simulink model "Validacion"  (R2022b)
settings: Solver=VariableStepAuto  StartTime=0.0  StopTime=10  RelTol=1e-3
values from neighbouring files (symbols this model uses):
  tt = tr-tr(1)    [LAB.m]
  ut = ur-u(pos(1)-1)    [LAB.m]
settings Model: Creator=emanu  LastModifiedBy=emanu

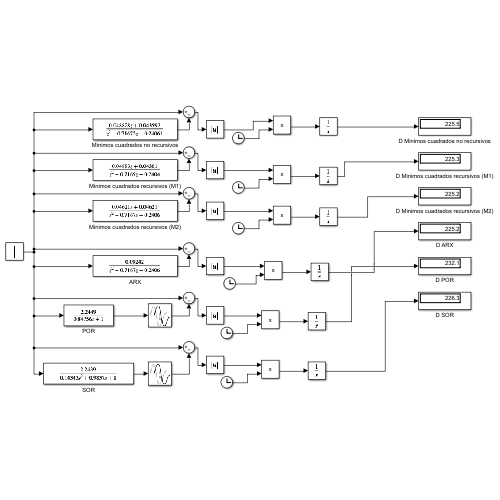
[thumbnail: Simulink's stored preview of the top-level diagram]
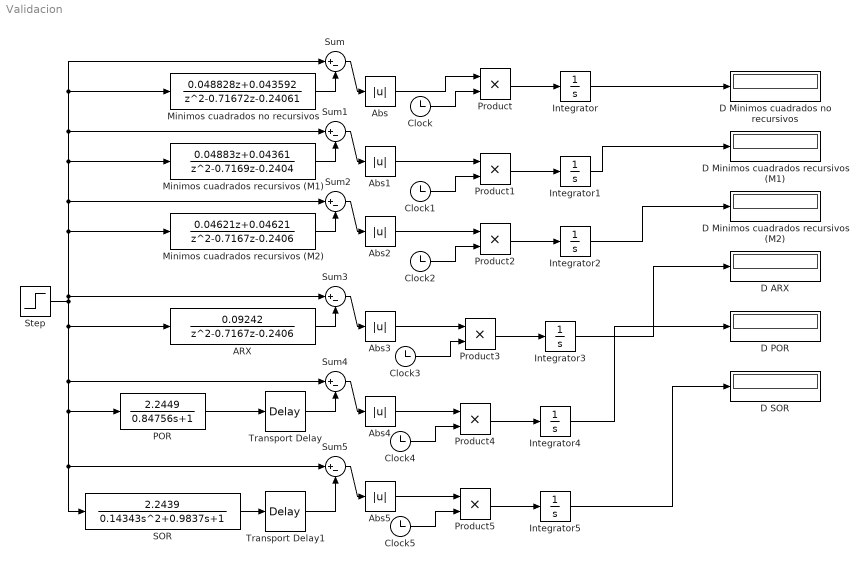
== system Validacion ==
  ARX : DiscreteTransferFcn  Numerator=[0 0.09242]  Denominator=[1 -0.7167 -0.2406]  SampleTime=tt(2)
  Abs{,1..5} (6 alike) : Abs  SaturateOnIntegerOverflow=off
  Clock{,1..5} (6 alike) : Clock
  D ARX : Display
  D Minimos cuadrados no recursivos : Display
  D Minimos cuadrados recursivos (M1) : Display
  D Minimos cuadrados recursivos (M2) : Display
  D POR : Display
  D SOR : Display
  Integrator{,1..5} (6 alike) : Integrator
  Minimos cuadrados no recursivos : DiscreteTransferFcn  Numerator=[0 0.048828 0.043592]  Denominator=[1 -0.71672 -0.24061]  SampleTime=tt(2)
  Minimos cuadrados recursivos (M1) : DiscreteTransferFcn  Numerator=[0 0.04883 0.04361]  Denominator=[1 -0.7169 -0.2404]  SampleTime=tt(2)
  Minimos cuadrados recursivos (M2) : DiscreteTransferFcn  Numerator=[0 0.04621 0.04621]  Denominator=[1 -0.7167 -0.2406]  SampleTime=tt(2)
  POR : TransferFcn  Numerator=[2.2449]  Denominator=[0.84756 1]
  Product{,1..5} (6 alike) : Product
  SOR : TransferFcn  Numerator=[2.2439]  Denominator=[0.14343 0.9837 1]
  Step : Step  After=ut(1)  SampleTime=0
  Sum{,1..5} (6 alike) : Sum  Inputs=|+-
  Transport Delay : TransportDelay  DelayTime=0.35428
  Transport Delay1 : TransportDelay
  wires:
  Clock/1 -> Product/2
  Product/1 -> Integrator/1
  Abs/1 -> Product/1
  Integrator/1 -> D Minimos cuadrados no recursivos/1
  Minimos cuadrados no recursivos/1 -> Sum/2
  Sum/1 -> Abs/1
  Minimos cuadrados recursivos (M1)/1 -> Sum1/2
  Sum1/1 -> Abs1/1
  Minimos cuadrados recursivos (M2)/1 -> Sum2/2
  Sum2/1 -> Abs2/1
  ARX/1 -> Sum3/2
  Sum3/1 -> Abs3/1
  Transport Delay/1 -> Sum4/2
  Sum4/1 -> Abs4/1
  Sum5/1 -> Abs5/1
  Integrator1/1 -> D Minimos cuadrados recursivos (M1)/1
  Clock1/1 -> Product1/2
  Product1/1 -> Integrator1/1
  Integrator2/1 -> D Minimos cuadrados recursivos (M2)/1
  Clock2/1 -> Product2/2
  Product2/1 -> Integrator2/1
  Integrator3/1 -> D ARX/1
  Clock3/1 -> Product3/2
  Product3/1 -> Integrator3/1
  Integrator4/1 -> D POR/1
  Clock4/1 -> Product4/2
  Product4/1 -> Integrator4/1
  Integrator5/1 -> D SOR/1
  Clock5/1 -> Product5/2
  Product5/1 -> Integrator5/1
  Abs1/1 -> Product1/1
  Abs2/1 -> Product2/1
  Abs3/1 -> Product3/1
  Abs4/1 -> Product4/1
  Abs5/1 -> Product5/1
  POR/1 -> Transport Delay/1
  SOR/1 -> Transport Delay1/1
  Step/1 -> Sum4/1, POR/1, Sum5/1, SOR/1, ARX/1, Sum3/1, Minimos cuadrados recursivos (M2)/1, Sum2/1, Minimos cuadrados recursivos (M1)/1, Sum1/1, Sum/1, Minimos cuadrados no recursivos/1
  Transport Delay1/1 -> Sum5/2
